simulink model "BJTModel"  (R2023b)
settings: Solver=ode1be  StartTime=0.0  StopTime=stop_time  FixedStep=Ts  RelTol=1e-3
values from neighbouring files (symbols this model uses):
  alpha_f = 236/(236+1)    (= 0.995780590717)    [dataset_generator.m]    (also in groundtruth_generator.m)
  alpha_r = 5.774/(5.774+1)    (= 0.852376734573)    [dataset_generator.m]    (also in groundtruth_generator.m)
  Is1 = 33.58e-15    (= 3.358e-14)    [dataset_generator.m]    (also in groundtruth_generator.m)
  Is2 = 33.58e-15    (= 3.358e-14)    [dataset_generator.m]    (also in groundtruth_generator.m)
  Rp1 = 1e11    (= 100000000000)    [dataset_generator.m]    (also in groundtruth_generator.m)
  Rp2 = 1e8    (= 100000000)    [dataset_generator.m]    (also in groundtruth_generator.m)
  Rs1 = 1e-5    (= 1e-05)    [dataset_generator.m]    (also in groundtruth_generator.m)
  Rs2 = 1e-5    (= 1e-05)    [dataset_generator.m]    (also in groundtruth_generator.m)
  Vt = 25.85e-3    (= 0.02585)    [dataset_generator.m]    (also in groundtruth_generator.m)
libraries: fl_lib x28, nesl_utility x8
settings Model: Creator=riccardo  LastModifiedBy=sebastian
settings SolverCC: AlgebraicLoopSolver=TrustRegion
settings DataIOCC: ReturnWorkspaceOutputsName=tp19cb4a2c_3148_4d73_bbe6_9ae95a49d26c
settings OptimizationCC: ReuseModelBlockBuffer=off
settings DebuggingCC: UnconnectedInputMsg=warning  UnconnectedOutputMsg=warning  UnconnectedLineMsg=warning
settings ModelReferenceCC: EnableRefExpFcnMdlSchedulingChecks=on

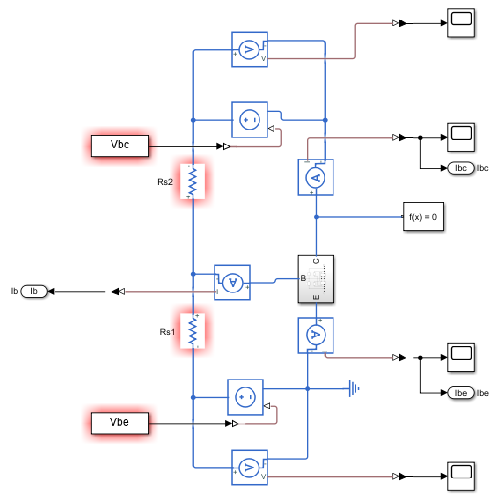
[thumbnail: Simulink's stored preview of the top-level diagram]
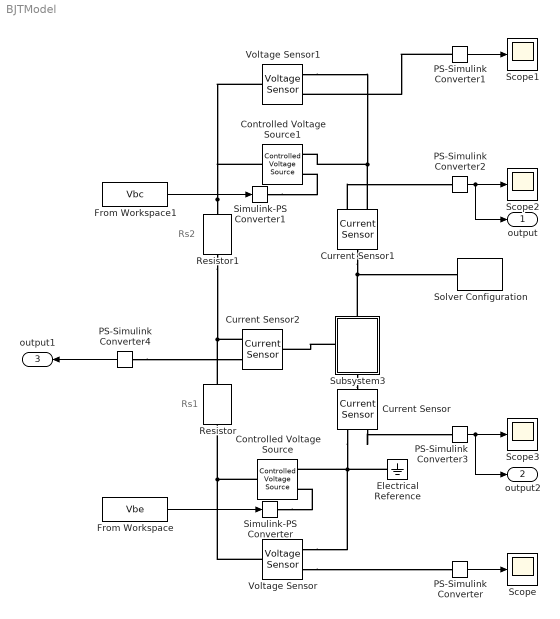
== system BJTModel ==
  note: Rs1
  note: Rs2
  Controlled Voltage Source : fl_lib/Electrical/Electrical Sources/Controlled Voltage Source
  Controlled Voltage Source1 : fl_lib/Electrical/Electrical Sources/Controlled Voltage Source
  Current Sensor : fl_lib/Electrical/Electrical Sensors/Current Sensor
  Current Sensor1 : fl_lib/Electrical/Electrical Sensors/Current Sensor
  Current Sensor2 : fl_lib/Electrical/Electrical Sensors/Current Sensor
  Electrical Reference : fl_lib/Electrical/Electrical Elements/Electrical Reference
  From Workspace : FromWorkspace  VariableName=Vbe
  From Workspace1 : FromWorkspace  VariableName=Vbc
  PS-Simulink Converter{,1..4} (5 alike) : nesl_utility/PS-Simulink Converter  PhysicalDomain=network_engine_domain  SubClassName=ps_output  LeftPortType=input  RightPortType=output  PseudoPeriodic=off  Frequencies=[]  VectorFormat=1-D array  Unit=inherit  AffineConversion=off
  Resistor : fl_lib/Electrical/Electrical Elements/Resistor  R=Rs1 Ohm  i_specify=off  i_priority=None  i=0 A  i_nominal_specify=off  i_nominal_unit=A  i_nominal_value=1  v_specify=off  v_priority=None  v=0 V  v_nominal_specify=off  v_nominal_unit=V  v_nominal_value=1
  Resistor1 : fl_lib/Electrical/Electrical Elements/Resistor  R=Rs2 Ohm  i_specify=off  i_priority=None  i=0 A  i_nominal_specify=off  i_nominal_unit=A  i_nominal_value=1  v_specify=off  v_priority=None  v=0 V  v_nominal_specify=off  v_nominal_unit=V  v_nominal_value=1
  Scope{,1..3} (4 alike) : Scope
  Simulink-PS Converter : nesl_utility/Simulink-PS Converter  PhysicalDomain=network_engine_domain  SubClassName=ps_input  LeftPortType=input  RightPortType=output  PseudoPeriodic=off  Frequencies=[]  NoiseDistribution=none  NoiseParameters=[]  Unit=1  AffineConversion=off  FilteringAndDerivatives=provide  SimscapeFilterOrder=1  InputFilterTimeConstant=0.001  UdotUserProvided=0
  Simulink-PS Converter1 : nesl_utility/Simulink-PS Converter  PhysicalDomain=network_engine_domain  SubClassName=ps_input  LeftPortType=input  RightPortType=output  PseudoPeriodic=off  Frequencies=[]  NoiseDistribution=none  NoiseParameters=[]  Unit=1  AffineConversion=off  FilteringAndDerivatives=provide  SimscapeFilterOrder=1  InputFilterTimeConstant=0.001  UdotUserProvided=0
  Solver Configuration : nesl_utility/Solver Configuration  PhysicalDomain=network_engine_domain  SubClassName=solver  LeftPortType=input  RightPortType=generic  Tones=[]  Harmonics=[]  SimulateNoise=off  Profile=off  UseLocalSampling=off  EnableSwitchedLinearOptims=on  FrequencyDomain=off  UseCCode=off  RelTol=0.001  AbsTol=1e-06  MinStep=1e-09  ToWorkspace=off  RevertToSquareIcSolve=off  NumHomotopyIterations=100  PhasorMode=off  PhasorModeNumHarmonics=1  ConsistencySolver=NEWTON_FTOL  IndexReductionMethod=DerivativeReplacement  DoDC=off  ResidualTolerance=1e-9  ConsistencyTolSource=GLOBAL  ConsistencyAbsTol=0.001  ConsistencyRelTol=0.001  ConsistencyTolFactor=0.001  UseLocalSolver=off  LocalSolverChoice=NE_BACKWARD_EULER_ADVANCER  ResolveIndetEquations=on  FunctionEvalNumThread=1  LocalSolverSampleTime=0.001  DoFixedCost=off  MaxNonlinIter=3  MaxModeIter=2  ComputeImpulses=off  ImpulseIterations=2  LinearAlgebra=auto  LinearAlgebraNumThread=0  EquationFormulation=NE_TIME_EF  DelaysMemoryBudget=1024  AutomaticFiltering=on  FilteringTimeConstant=0.001  PartitionStorageMethod=AS_NEEDED  PartitionMemoryBudget=1024  PartitionMethod=ROBUST  MultibodyUseLocalSolver=off  MultibodyLocalSolverChoice=ODE1  MultibodyLocalSolverSampleTime=0.001
  Subsystem3 : Subsystem
      settings: PortSchema="{\"entries\":[{\"content\":{\"sides\":[{\"content\":{\"connectorIds\":[\"LConn1\"]},\"type\":\"ConnectorPlacement.EquallySpacedRectSide\",\"uuid\":\"e7d2ad01-b729-4278-a2af-615928332c77\"},{\"content\":{\"side\":\"RIGHT\"},\"type\":\"ConnectorPlacement.EquallySpacedRectSide\",\"uuid\":\"6c8f5083-1d74-476b-8fc8-74f7e6a90163\"},{\"content\":{\"connectorIds\":[\"LConn2\"],\"side\":\"TOP\"},\"type\":\"ConnectorPlacement.EquallySpacedRectSide\",\"uuid\":\"cf8d2faf-1e25-415e-bca0-3701d5262d4d\"},{\"content\":{\"connectorIds\":[\"RConn1\"],\"side\":\"BOTTOM\"},\"type\":\"ConnectorPlacement.EquallySpacedRectSide\",\"uuid\":\"80ad8aee-c458-4554-96ef-dc25eb201335\"}]},\"type\":\"ConnectorPlacement.EquallySpacedConnector\",\"uuid\":\"23596b54-1579-47cb-b7ec-00e276fa3e81\"}],\"packageUris\":[\"http://schema.mathworks.com/mf0/Connector/R2020b\"],\"version\":\"1.0\"}"
  Voltage Sensor : fl_lib/Electrical/Electrical Sensors/Voltage Sensor
  Voltage Sensor1 : fl_lib/Electrical/Electrical Sensors/Voltage Sensor
  output : Outport  SignalName=Ibc
  output2 : Outport  Port=2  SignalName=Ibe
  output1 : Outport  Port=3  SignalName=Ib
  wires:
  PS-Simulink Converter/1 -> Scope/1
  PS-Simulink Converter1/1 -> Scope1/1
  PS-Simulink Converter2/1 -> output/1, Scope2/1
  PS-Simulink Converter3/1 -> output2/1, Scope3/1
  From Workspace/1 -> Simulink-PS Converter/1
  From Workspace1/1 -> Simulink-PS Converter1/1
  PS-Simulink Converter4/1 -> output1/1
  connections:
  Current Sensor1/LConn1 -- Subsystem3/LConn2 -- Solver Configuration/RConn1
  Voltage Sensor/LConn1 -- Controlled Voltage Source/LConn1 -- Resistor/RConn1
  Voltage Sensor/RConn2 -- Controlled Voltage Source/RConn2 -- Electrical Reference/LConn1 -- Current Sensor/RConn2
  Voltage Sensor/RConn1 -- PS-Simulink Converter/LConn1
  Resistor/LConn1 -- Current Sensor2/RConn2 -- Resistor1/LConn1
  Resistor1/RConn1 -- Controlled Voltage Source1/LConn1 -- Voltage Sensor1/LConn1
  PS-Simulink Converter1/LConn1 -- Voltage Sensor1/RConn1
  Voltage Sensor1/RConn2 -- Current Sensor1/RConn2 -- Controlled Voltage Source1/RConn2
  Current Sensor1/RConn1 -- PS-Simulink Converter2/LConn1
  Current Sensor/RConn1 -- PS-Simulink Converter3/LConn1
  Simulink-PS Converter/RConn1 -- Controlled Voltage Source/RConn1
  Simulink-PS Converter1/RConn1 -- Controlled Voltage Source1/RConn1
  PS-Simulink Converter4/LConn1 -- Current Sensor2/RConn1
  Subsystem3/RConn1 -- Current Sensor/LConn1
  Subsystem3/LConn1 -- Current Sensor2/LConn1

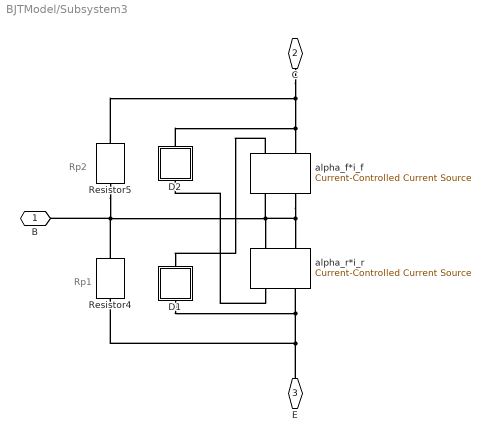
== system BJTModel/Subsystem3 ==
  note: Rp1
  note: Rp2
  D1 : Subsystem
  D2 : Subsystem
  Resistor4 : fl_lib/Electrical/Electrical Elements/Resistor  R=Rp1 Ohm  i_specify=off  i_priority=None  i=0 A  i_nominal_specify=off  i_nominal_unit=A  i_nominal_value=1  v_specify=off  v_priority=None  v=0 V  v_nominal_specify=off  v_nominal_unit=V  v_nominal_value=1
  Resistor5 : fl_lib/Electrical/Electrical Elements/Resistor  R=Rp2 Ohm  i_specify=off  i_priority=None  i=0 A  i_nominal_specify=off  i_nominal_unit=A  i_nominal_value=1  v_specify=off  v_priority=None  v=0 V  v_nominal_specify=off  v_nominal_unit=V  v_nominal_value=1
  alpha_f*i_f : fl_lib/Electrical/Electrical Sources/Current-Controlled Current Source  K=alpha_f  i1_specify=off  i1_priority=High  i1=0 A  i1_nominal_specify=off  i1_nominal_unit=A  i1_nominal_value=1  i2_specify=off  i2_priority=High  i2=0 A  i2_nominal_specify=off  i2_nominal_unit=A  i2_nominal_value=1
      settings: InternalSimscapePortConfiguration="{\"Bottom\":[],\"Left\":[{\"id\":\"p1\",\"label\":\"+\",\"type\":\"foundation.electrical.electrical\"},{\"id\":\"head\",\"label\":\"\",\"type\":\"foundation.electrical.electrical\"}],\"Right\":[{\"id\":\"n1\",\"label\":\"-\",\"type\":\"foundation.electrical.electrical\"},{\"id\":\"tail\",\"label\":\"\",\"type\":\"foundation.electrical.electrical\"}],\"Top\":[]}"
  alpha_r*i_r : fl_lib/Electrical/Electrical Sources/Current-Controlled Current Source  K=alpha_r  i1_specify=off  i1_priority=High  i1=0 A  i1_nominal_specify=off  i1_nominal_unit=A  i1_nominal_value=1  i2_specify=off  i2_priority=High  i2=0 A  i2_nominal_specify=off  i2_nominal_unit=A  i2_nominal_value=1
      settings: InternalSimscapePortConfiguration="{\"Bottom\":[],\"Left\":[{\"id\":\"p1\",\"label\":\"+\",\"type\":\"foundation.electrical.electrical\"},{\"id\":\"head\",\"label\":\"\",\"type\":\"foundation.electrical.electrical\"}],\"Right\":[{\"id\":\"n1\",\"label\":\"-\",\"type\":\"foundation.electrical.electrical\"},{\"id\":\"tail\",\"label\":\"\",\"type\":\"foundation.electrical.electrical\"}],\"Top\":[]}"
  B : PMIOPort  Side=Left
  C : PMIOPort  Port=2  Side=Left
  E : PMIOPort  Port=3  Side=Right
  connections:
  D1/RConn1 -- alpha_r*i_r/RConn2 -- E/RConn1 -- Resistor4/RConn1
  D2/RConn1 -- alpha_f*i_f/RConn2 -- C/RConn1 -- Resistor5/LConn1
  alpha_f*i_f/LConn1 -- alpha_r*i_r/LConn1 -- alpha_r*i_r/LConn2 -- alpha_f*i_f/LConn2 -- Resistor4/LConn1 -- B/RConn1 -- Resistor5/RConn1
  alpha_f*i_f/RConn1 -- D1/LConn1
  alpha_r*i_r/RConn1 -- D2/LConn1

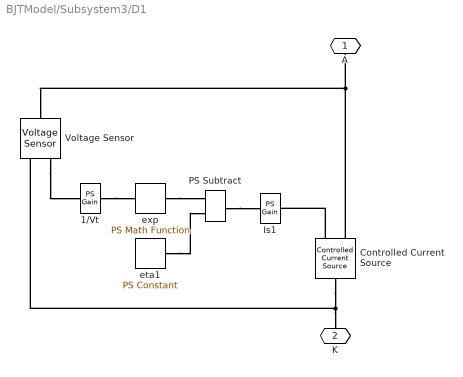
== system BJTModel/Subsystem3/D1 ==
  1/Vt : fl_lib/Physical Signals/Functions/PS Gain  gain=1/Vt 1/V
  Controlled Current Source : fl_lib/Electrical/Electrical Sources/Controlled Current Source
  Is1 : fl_lib/Physical Signals/Functions/PS Gain  gain=Is1 A
  PS Subtract : fl_lib/Physical Signals/Functions/PS Subtract
  Voltage Sensor : fl_lib/Electrical/Electrical Sensors/Voltage Sensor
  eta1 : fl_lib/Physical Signals/Sources/PS Constant  constant=N_f
  exp : fl_lib/Physical Signals/Functions/PS Math Function  fcn_choice=3  v=1
  A : PMIOPort  Side=Left
  K : PMIOPort  Port=2  Side=Right
  connections:
  K/RConn1 -- Controlled Current Source/LConn1 -- Voltage Sensor/RConn2
  Controlled Current Source/RConn1 -- Is1/RConn1
  PS Subtract/RConn1 -- Is1/LConn1
  eta1/RConn1 -- PS Subtract/LConn2
  exp/RConn1 -- PS Subtract/LConn1
  1/Vt/RConn1 -- exp/LConn1
  Voltage Sensor/RConn1 -- 1/Vt/LConn1
  A/RConn1 -- Voltage Sensor/LConn1 -- Controlled Current Source/RConn2

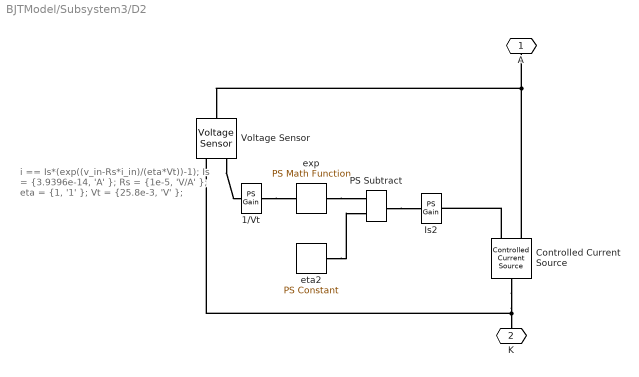
== system BJTModel/Subsystem3/D2 ==
  note: i == Is*(exp((v_in-Rs*i_in)/(eta*Vt))-1);
      | Is = {3.9396e-14, 'A' };
      | Rs = {1e-5, 'V/A' };
      | eta = {1, '1' };
      | Vt = {25.8e-3, 'V' };
  1/Vt : fl_lib/Physical Signals/Functions/PS Gain  gain=1/Vt 1/V
  Controlled Current Source : fl_lib/Electrical/Electrical Sources/Controlled Current Source
  Is2 : fl_lib/Physical Signals/Functions/PS Gain  gain=Is2 A
  PS Subtract : fl_lib/Physical Signals/Functions/PS Subtract
  Voltage Sensor : fl_lib/Electrical/Electrical Sensors/Voltage Sensor
  eta2 : fl_lib/Physical Signals/Sources/PS Constant  constant=N_r
  exp : fl_lib/Physical Signals/Functions/PS Math Function  fcn_choice=3  v=1
  A : PMIOPort  Side=Left
  K : PMIOPort  Port=2  Side=Right
  connections:
  Controlled Current Source/RConn2 -- Voltage Sensor/LConn1 -- A/RConn1
  Voltage Sensor/RConn1 -- 1/Vt/LConn1
  1/Vt/RConn1 -- exp/LConn1
  exp/RConn1 -- PS Subtract/LConn1
  eta2/RConn1 -- PS Subtract/LConn2
  PS Subtract/RConn1 -- Is2/LConn1
  Controlled Current Source/RConn1 -- Is2/RConn1
  K/RConn1 -- Voltage Sensor/RConn2 -- Controlled Current Source/LConn1
